simulink model "ICUB27_HEAD"  (R2021b)
settings: Solver=VariableStepAuto  StartTime=0.0  StopTime=10.0  RelTol=1e-3
model workspace: external: MATLAB File C:\Users\mfussi\iit\ergocub\ergocub-design-head\neck-mechanism-study\models\resources_head_icub\ICUB27_HEAD_DataFile.m (data not in the file)
undefined symbols (not defined in the file): headData, X, Y, Z
libraries: sm_lib x9, nesl_utility x1
settings Model: Creator=mfussi  LastModifiedBy=mfussi

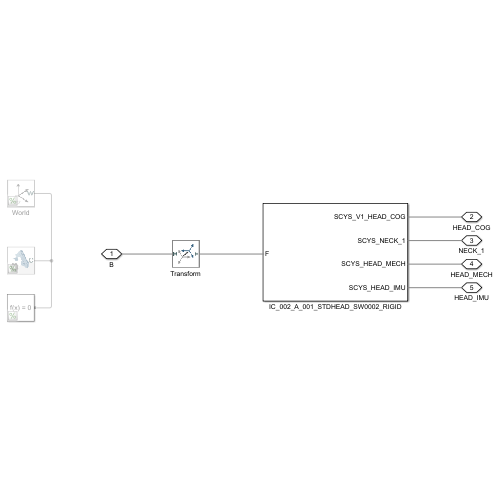
[thumbnail: Simulink's stored preview of the top-level diagram]
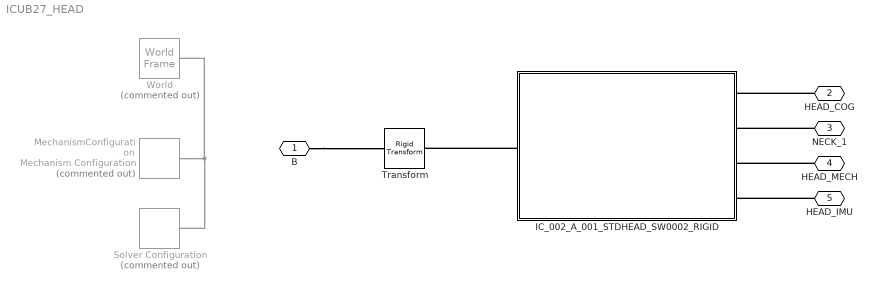
== system ICUB27_HEAD ==
  IC_002_A_001_STDHEAD_SW0002_RIGID : Subsystem
  MechanismConfiguration : sm_lib/Utilities/Mechanism Configuration  Commented=on  UniformGravity=Constant  GravityVector=[0 -9.80665 0]  GravityUnits=m/s^2  LinearizationDelta=0.001  JointModeTransitionNonlinearIterations=2
  Solver Configuration : nesl_utility/Solver Configuration  Commented=on  PhysicalDomain=network_engine_domain  SubClassName=solver  LeftPortType=input  RightPortType=generic  Tones=[]  Harmonics=[]  SimulateNoise=off  Profile=off  UseLocalSampling=off  EnableSwitchedLinearOptims=on  FrequencyDomain=off  UseCCode=off  RelTol=0.001  AbsTol=1e-06  MinStep=1e-09  ToWorkspace=off  RevertToSquareIcSolve=off  NumHomotopyIterations=100  PhasorMode=off  PhasorModeNumHarmonics=1  DoDC=off  ResidualTolerance=1e-09  UseLocalSolver=off  LocalSolverChoice=NE_BACKWARD_EULER_ADVANCER  LocalSolverSampleTime=0.001  DoFixedCost=off  MaxNonlinIter=3  MaxModeIter=2  ComputeImpulses=off  ImpulseIterations=2  LinearAlgebra=auto  EquationFormulation=NE_TIME_EF  DelaysMemoryBudget=1024  AutomaticFiltering=on  FilteringTimeConstant=0.001  PartitionStorageMethod=AS_NEEDED  PartitionMemoryBudget=1024  PartitionMethod=ROBUST
      settings: SourceProductBaseCode=PW,SS
  Transform : sm_lib/Frames and Transforms/Rigid Transform  TranslationMethod=Cartesian  TranslationStandardOffset=0  TranslationLengthUnit=mm  TranslationStandardAxis=+Z  TranslationCartesianOffset=headData.RigidTransform(5).translation  TranslationROffset=0  TranslationROffsetUnits=m  TranslationZOffset=0  TranslationZOffsetUnits=m  TranslationThetaOffset=0  TranslationThetaOffsetUnits=deg  RotationMethod=ArbitraryAxis  RotationAngleUnits=rad  RotationStandardAxis=+Z  RotationAngle=headData.RigidTransform(5).angle  RotationArbitraryAxis=headData.RigidTransform(5).axis  FollAlignAxisA=+X  BaseAlignAxisA=+Y  FollAlignAxisB=+Y  BaseAlignAxisB=+Z  RotationSequenceAxes=FollowerAxes  RotationSequence=XYX  RotationSequenceAngles=[0 0 0]  RotationSequenceAnglesUnits=deg  RotationMatrix=[1 0 0; 0 1 0; 0 0 1]
  World : sm_lib/Frames and Transforms/World Frame  Commented=on
  B : PMIOPort  Side=Left
  HEAD_COG : PMIOPort  Port=2  Side=Left
  NECK_1 : PMIOPort  Port=3  Side=Left
  HEAD_MECH : PMIOPort  Port=4  Side=Left
  HEAD_IMU : PMIOPort  Port=5  Side=Left
  connections:
  MechanismConfiguration/RConn1 -- World/RConn1 -- Solver Configuration/RConn1
  IC_002_A_001_STDHEAD_SW0002_RIGID/LConn1 -- Transform/RConn1
  B/RConn1 -- Transform/LConn1
  HEAD_COG/RConn1 -- IC_002_A_001_STDHEAD_SW0002_RIGID/RConn1
  NECK_1/RConn1 -- IC_002_A_001_STDHEAD_SW0002_RIGID/RConn2
  HEAD_MECH/RConn1 -- IC_002_A_001_STDHEAD_SW0002_RIGID/RConn3
  HEAD_IMU/RConn1 -- IC_002_A_001_STDHEAD_SW0002_RIGID/RConn4

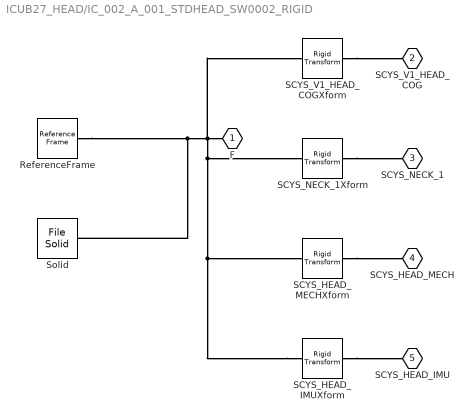
== system ICUB27_HEAD/IC_002_A_001_STDHEAD_SW0002_RIGID ==
  ReferenceFrame : sm_lib/Frames and Transforms/Reference Frame
  SCYS_HEAD_IMUXform : sm_lib/Frames and Transforms/Rigid Transform  TranslationMethod=Cartesian  TranslationStandardOffset=0  TranslationLengthUnit=mm  TranslationStandardAxis=+Z  TranslationCartesianOffset=headData.RigidTransform(2).translation  TranslationROffset=0  TranslationROffsetUnits=m  TranslationZOffset=0  TranslationZOffsetUnits=m  TranslationThetaOffset=0  TranslationThetaOffsetUnits=deg  RotationMethod=ArbitraryAxis  RotationAngleUnits=rad  RotationStandardAxis=+Z  RotationAngle=headData.RigidTransform(2).angle  RotationArbitraryAxis=headData.RigidTransform(2).axis  FollAlignAxisA=+X  BaseAlignAxisA=+Y  FollAlignAxisB=+Y  BaseAlignAxisB=+Z  RotationSequenceAxes=FollowerAxes  RotationSequence=XYX  RotationSequenceAngles=[0 0 0]  RotationSequenceAnglesUnits=deg  RotationMatrix=[1 0 0; 0 1 0; 0 0 1]
  SCYS_HEAD_MECHXform : sm_lib/Frames and Transforms/Rigid Transform  TranslationMethod=Cartesian  TranslationStandardOffset=0  TranslationLengthUnit=mm  TranslationStandardAxis=+Z  TranslationCartesianOffset=headData.RigidTransform(4).translation  TranslationROffset=0  TranslationROffsetUnits=m  TranslationZOffset=0  TranslationZOffsetUnits=m  TranslationThetaOffset=0  TranslationThetaOffsetUnits=deg  RotationMethod=ArbitraryAxis  RotationAngleUnits=rad  RotationStandardAxis=+Z  RotationAngle=headData.RigidTransform(4).angle  RotationArbitraryAxis=headData.RigidTransform(4).axis  FollAlignAxisA=+X  BaseAlignAxisA=+Y  FollAlignAxisB=+Y  BaseAlignAxisB=+Z  RotationSequenceAxes=FollowerAxes  RotationSequence=XYX  RotationSequenceAngles=[0 0 0]  RotationSequenceAnglesUnits=deg  RotationMatrix=[1 0 0; 0 1 0; 0 0 1]
  SCYS_NECK_1Xform : sm_lib/Frames and Transforms/Rigid Transform  TranslationMethod=Cartesian  TranslationStandardOffset=0  TranslationLengthUnit=mm  TranslationStandardAxis=+Z  TranslationCartesianOffset=headData.RigidTransform(3).translation  TranslationROffset=0  TranslationROffsetUnits=m  TranslationZOffset=0  TranslationZOffsetUnits=m  TranslationThetaOffset=0  TranslationThetaOffsetUnits=deg  RotationMethod=ArbitraryAxis  RotationAngleUnits=rad  RotationStandardAxis=+Z  RotationAngle=headData.RigidTransform(3).angle  RotationArbitraryAxis=headData.RigidTransform(3).axis  FollAlignAxisA=+X  BaseAlignAxisA=+Y  FollAlignAxisB=+Y  BaseAlignAxisB=+Z  RotationSequenceAxes=FollowerAxes  RotationSequence=XYX  RotationSequenceAngles=[0 0 0]  RotationSequenceAnglesUnits=deg  RotationMatrix=[1 0 0; 0 1 0; 0 0 1]
  SCYS_V1_HEAD_COGXform : sm_lib/Frames and Transforms/Rigid Transform  TranslationMethod=Cartesian  TranslationStandardOffset=0  TranslationLengthUnit=mm  TranslationStandardAxis=+Z  TranslationCartesianOffset=headData.RigidTransform(1).translation  TranslationROffset=0  TranslationROffsetUnits=m  TranslationZOffset=0  TranslationZOffsetUnits=m  TranslationThetaOffset=0  TranslationThetaOffsetUnits=deg  RotationMethod=ArbitraryAxis  RotationAngleUnits=rad  RotationStandardAxis=+Z  RotationAngle=headData.RigidTransform(1).angle  RotationArbitraryAxis=headData.RigidTransform(1).axis  FollAlignAxisA=+X  BaseAlignAxisA=+Y  FollAlignAxisB=+Y  BaseAlignAxisB=+Z  RotationSequenceAxes=FollowerAxes  RotationSequence=XYX  RotationSequenceAngles=[0 0 0]  RotationSequenceAnglesUnits=deg  RotationMatrix=[1 0 0; 0 1 0; 0 0 1]
  Solid : sm_lib/Body Elements/File Solid  ExtGeomFileName=ic_002_a_001_stdhead_sw0002_prt.step  UnitType=FromFile  ExtGeomFileUnits=m  StepReaderType=HEX  ExportConvexHullGeometry=off  InertiaType=Custom  Mass=headData.Solid(1).mass  MassUnits=kg  CenterOfMass=headData.Solid(1).CoM  CenterOfMassUnits=mm  MomentsOfInertia=headData.Solid(1).MoI  MomentsOfInertiaUnits=kg*mm^2  ProductsOfInertia=headData.Solid(1).PoI  ProductsOfInertiaUnits=kg*mm^2  BasedOnType=DensityFromFile  Density=1000  DensityUnits=kg/m^3  DoExposeReferenceFrame=on  SerializedFrames=<Frames/>  GraphicType=FromGeometry  MarkerShape=Sphere  MarkerSize=10  GraphicVisPropType=SimpleVisualProperties  GraphicDiffuseColor=headData.Solid(1).color  GraphicSpecularColor=[0.5 0.5 0.5 1.0]  GraphicAmbientColor=[0.15 0.15 0.15 1.0]  GraphicEmissiveColor=[0.0 0.0 0.0 1.0]  GraphicShininess=75  GraphicOpacity=headData.Solid(1).opacity
  F : PMIOPort  Side=Left
  SCYS_V1_HEAD_COG : PMIOPort  Port=2  Side=Right
  SCYS_NECK_1 : PMIOPort  Port=3  Side=Right
  SCYS_HEAD_MECH : PMIOPort  Port=4  Side=Right
  SCYS_HEAD_IMU : PMIOPort  Port=5  Side=Right
  connections:
  SCYS_HEAD_IMUXform/LConn1 -- ReferenceFrame/RConn1 -- Solid/RConn1 -- SCYS_V1_HEAD_COGXform/LConn1 -- F/RConn1 -- SCYS_NECK_1Xform/LConn1 -- SCYS_HEAD_MECHXform/LConn1
  SCYS_V1_HEAD_COGXform/RConn1 -- SCYS_V1_HEAD_COG/RConn1
  SCYS_HEAD_IMUXform/RConn1 -- SCYS_HEAD_IMU/RConn1
  SCYS_NECK_1Xform/RConn1 -- SCYS_NECK_1/RConn1
  SCYS_HEAD_MECHXform/RConn1 -- SCYS_HEAD_MECH/RConn1
